simulink model "Clutchless_P2_Parallel_ETE"  (R2017b)
settings: Solver=FixedStepAuto  StartTime=0.0  StopTime=length(Speed)  FixedStep=0.01  MaxStep=0.01  RelTol=1e-3  EnableMultiTasking=on
PostLoadFcn:
  | , if any(exist('dsrtsu_mdlpostloadfcn', 'file') == [2, 3, 6]), try dsrtsu_mdlpostloadfcn('Execute', bdroot); catch fprintf('Error in PostLoadFcn (dsrtsu_mdlpostloadfcn) for model "%s":\n %s\n', bdroot, lasterr); end, end,
undefined symbols (not defined in the file): ABSEnable, Actuators, air, APP1_OOR, APP2_OOR, APP_Mismatch, Brk_Flt, cal, ClutchEngag, Clutchless_HSC_ETE, CS_On_Control, Driver, eng, Engine, EngOverTemp, ENGTRQ_MSMCH_Degraded_CP, ENGTRQ_MSMCH_ErrCritical_CP, ENGTRQ_MSMCH_LimpHome_CP, EngTrqMismatch, env, ess, ESSOverTemp, gb, KeyPos_Flt, KeyPosition, lib_Actuators, lib_Clutchless_HSC_ETE, lib_Driver, lib_EMachine_2017a, lib_Sensors_2017a, LossCAN, Machine, max_vehicle_rad_air_flow, MCUOverTemp, mot, MotDirMismatch, MotOverTemp, MotTrqMismatch, mph2ms, PRNDL_Flt, RegenBrkDisable, RegenFault, Sensors, ShiftLeverPosition, Speed, SW_CS_ON, SW_Engine_ON, t_amb, time, tloop
libraries: simulink x97, Pneumatic_lib x11, nesl_utility x9, EC2_libraries x7, powerlib_meascontrol x2, CalculationGallon x1, lib_Chassis x1, lib_DCDC x1, lib_Differential x1, lib_HVESS x1, fl_lib x1, lib_OBC x1
(part 9 of 9)

== stateflow chart Clutchless_P2_Parallel_ETE/Camaro Plant Model/ICE Simple1/Engine Plant Modified/Core Engine/Crank Process ==
  state Starter_Crank
    du:
    EngActTrq = function(EngSpd_RPM);
  state Eng_Off
    du:
    EngActTrq = 0;
  state Eng_Combustion
    du:
    EngActTrq = 100;
  state CrankTrq = function(EngSpd) [function]
  state Eng_Run
    du:
    EngActTrq = EngBrkTrq;
  (default) -> Eng_Off
  Eng_Off -> Starter_Crank : [EngCrankCmd]
  Starter_Crank -> Eng_Off [order 2] : [!EngCrankCmd]
  Eng_Run -> Eng_Off : [AvlblFuel <= 0.01|| EngShutdown == 1]
  Starter_Crank -> Eng_Combustion [order 1] : [AvlblFuel >= 0.1]
  Eng_Combustion -> Eng_Run : [EngRunAtv]
  data: CrankTrq function_output; EngSpd function_input; EngRunAtv input boolean; AvlblFuel input double; EngActTrq output double; EngCrankCmd input boolean; EngBrkTrq input double; EngSpd_RPM input double; EngShutdown input boolean

== stateflow chart Clutchless_P2_Parallel_ETE/Camaro Plant Model/ICE Simple1/Soft ECM/ECM_RollingAliveCnt/Rolling Alive Counter ==
  state RollingAliveCounter
    state Count1
      en: RollingAliveCnt = 0;
    state Count2
      en: RollingAliveCnt = 1;
    state Count3
      en: RollingAliveCnt = 2;
    state Count4
      en: RollingAliveCnt = 3;
    (default) -> Count1
    Count4 -> Count1 : after(0.01,sec)
    Count1 -> Count2 : after(0.01,sec)
    Count2 -> Count3 : after(0.01,sec)
    Count3 -> Count4 : after(0.01,sec)
  data: RollingAliveCnt output int8 =0

== stateflow chart Clutchless_P2_Parallel_ETE/Camaro Plant Model/ICE Simple1/Soft ECM/Logic ==
  state Eng_Crank
    en:
    EngCrankCmd = 1;
    FuelPumpEnable = 1;
    EngShutdown = 0;
  state Eng_Off
    en:
    EngRunAtv = 0;
    EngCrankCmd = 0;
    ThrottleCmd = 0;
    FuelPumpEnable = 0;
  state Eng_On
    en:
    EngRunAtv = 1;
    EngCrankCmd = 0;
    du:
    ThrottleCmd = APP2TP(drvAPP,EngSpd_RPM);
  state TP = APP2TP(APP,EngSpd) [function]
  (default) -> Eng_Off
  Eng_Off -> Eng_Crank : [SysPwrMd == 3]
  Eng_Crank -> Eng_Off [order 2] : [SysPwrMd < 3]
  Eng_On -> Eng_Off : [SysPwrMd < 2 || EngSpd_RPM < 500]
      | {EngShutdown = 1; }
  Eng_Crank -> Eng_On [order 1] : [EngSpd_RPM >= 580]
  data: TP function_output; APP function_input; EngSpd function_input; drvAPP input; ThrottleCmd output double; EngCrankCmd output boolean; SysPwrMd input int8; ShftLvrPos input int8; EngSpd_RPM input double; VehSpdAvgDrvn input double; EngRunAtv output boolean; FuelPumpEnable output double; EngShutdown output boolean

== stateflow chart Clutchless_P2_Parallel_ETE/Clutchless_HSC_ETE/HSC/Powertrain Manager/HV Manager1/Inverter Manager/MCU_Manager  ==
  state MCU_Initialization
    state MCU_Request_Standby
      en:
      MCU_State = 1;
      RequestedStateINV = 3;
      CAN_Activation = 1;
    state Power_Off_INVCON
      entry:
      MCU_State = 0;
      INVCON_Power =0;
    state Power_On_INVCON
      en:MCU_State = 2;
      INVCON_Power =1;
    state HV_CAN_Actuation_Fault
      en:
      MCU_State = -1;
      CAN_Activation = 0;
    state INVCON_Power_Fault
      en:
      MCU_State = -2;
      INVCON_Power =0;
      CAN_Activation = 0;
    Power_Off_INVCON -> (junction 18) : {Timer=0;}
    (junction 18) -> MCU_Request_Standby [order 1] : [HVCAN_State]
    HV_CAN_Actuation_Fault -> (junction 18) : [HVCAN_State]
    (junction 18) -> HV_CAN_Actuation_Fault [order 2] : after(3,sec)
    (default) -> Power_Off_INVCON
    MCU_Request_Standby -> Power_On_INVCON : [HV_State == 9]
    Power_On_INVCON -> INVCON_Power_Fault : after(3,sec)
        | [INV_State ~= 3]
  state MCU_TorqueMode
    state MCU_Enable
      en:MCU_State = 4;
      RequestedStateINV = 8;
      during: Timer = Timer + 1;
    state MCU_Ready
      en:
      MCU_State = 3;
    state MCU_Running
      en:
      MCU_State =5;
    state TorqueCommand_Reject_Fault
      en:
      MCU_State = -3;
      RequestedStateINV = 3;
    state MCU_Stop
      en:
      MCU_State = 6;
      RequestedStateINV = 3;
    (default) -> MCU_Ready
    MCU_Enable -> (junction 35)
    (junction 35) -> MCU_Running [order 1] : [INV_State == 8]
    MCU_Ready -> MCU_Enable : [EnableInverter]
        | {Timer = 0;}
    (junction 35) -> TorqueCommand_Reject_Fault [order 2] : after(10,sec)
    MCU_Running -> MCU_Stop : [~ReadyToDrive]
  state MCU_Shutdown
    state MCU_Off
      en:
      MCU_State = 11;
      RequestedStateINV = 3;
      INVCON_Power = 0;
    state MCU_Dschrg
      en:
      MCU_State = 10;
      RequestedStateINV = 14;
    state MCU_RdyForShtDwn
      en:
      MCU_State = 9;
    (default) -> MCU_RdyForShtDwn
    MCU_RdyForShtDwn -> MCU_Dschrg : [~EnableInverter]
        | {Timer = 0;}
    MCU_Dschrg -> MCU_Off : [INV_State == 14 && LinkVoltage<60]
  (default) -> MCU_Initialization
  MCU_Shutdown -> MCU_Initialization : [KeyPos>= 1]
  MCU_Initialization -> MCU_Shutdown [order 2] : [ReadyToCharge]
  MCU_TorqueMode -> MCU_Initialization [order 1] : [INV_State == 14]
  MCU_Initialization -> MCU_TorqueMode [order 1] : [INV_State == 3 && INVCON_Power_Feedback && ReadyToDrive]
  MCU_TorqueMode -> MCU_Shutdown [order 2] : [INV_State == 3 && ~ReadyToDrive]
  data: ReadyToDrive input boolean; ReadyToCharge input; HV_State input; HVCAN_State input boolean; INVCON_Power_Feedback input; KeyPos input; LinkVoltage input; INV_State input; INV_CurrentHV input; Timer local double; MCU_State output; EnableInverter input boolean; ShutdownCurrent input; INVCON_Power output double; RequestedStateINV output; CAN_Activation output

== matlab function Clutchless_P2_Parallel_ETE/Camaro Plant Model/E-Machine/Soft MCU/diff_INV_state1 ==
  data: u input; y output
function y = fcn(u)
if(u == 0) %when inverter is in standby state
    y = 0;
elseif(u == 1) %when inverter is in torque control state
    y = 1;
elseif(u==2) %when invertor is in error state
    y = 0;
else
    y = 0;
end

== stateflow chart Clutchless_P2_Parallel_ETE/Clutchless_HSC_ETE/HSC/Camaro Fault Detection/Signal Diagnostic/ESS Signal Diagnostic/ESS SOC Validity Check/essSOC_0_1Range ==
  state aboveMax
    en: essSOCRange=3;
  state NormalRange
    en: essSOCRange=2;
  state LowRange
    en:essSOCRange=1;
  state BelowNormal
    en: essSOCRange=0;
  aboveMax -> NormalRange : [signalValue<0.95]
  NormalRange -> aboveMax [order 1] : [signalValue>=0.95]
  NormalRange -> NormalRange [order 3] : [clearFaults==1]
      | {essSOCRange=2;}
  (default) -> NormalRange
  LowRange -> NormalRange [order 1] : [signalValue>0.3]
  NormalRange -> LowRange [order 2] : [signalValue<=0.3&&signalValue>0.15]
  LowRange -> BelowNormal [order 2] : [signalValue<=0.15]
  BelowNormal -> LowRange : [signalValue>0.15]
  data: clearFaults input; signalValue input; data local; essSOCRange output

== stateflow chart Clutchless_P2_Parallel_ETE/Clutchless_HSC_ETE/HSC/Camaro Fault Detection/Signal Diagnostic/ESS Signal Diagnostic/ESS Temp Validity Check/essTsignalRange ==
  state AboveMax
    en: essTempRange=4;
  state HighRange
    en: essTempRange=3;
  state NormalRange
    en: essTempRange=2;
  state LowRange
    en:essTempRange=1;
  state BelowNormal
    en: essTempRange=0;
  HighRange -> AboveMax [order 2] : [signalValue>55]
  AboveMax -> HighRange : [signalValue<55]
  HighRange -> NormalRange [order 1] : [signalValue<=30]
  NormalRange -> HighRange [order 1] : [signalValue>32]
  NormalRange -> NormalRange [order 3] : [clearFaults==1]
      | {essTempRange=2;}
  (default) -> NormalRange
  LowRange -> NormalRange [order 1] : [signalValue>=30]
  NormalRange -> LowRange [order 2] : [signalValue<0 ]
  LowRange -> BelowNormal [order 2] : [signalValue<-28]
  BelowNormal -> LowRange : [signalValue>28]
  data: clearFaults input; signalValue input; essTempRange output; data local

== stateflow chart Clutchless_P2_Parallel_ETE/Clutchless_HSC_ETE/HSC/Camaro Fault Detection/Signal Diagnostic/ESS Signal Diagnostic/Rolling Alive Counter Detection/Chart ==
  state Off
    en:flag=0;
  state Alive
    en:flag=1;
  state Dead
    en:flag=0;
  Alive -> Alive [order 1] : after(CycleTime-tloop,sec)
      | [PulseDetect==1]
  (default) -> Off
  Off -> Alive : [PulseDetect==1]
  Alive -> Dead [order 2] : after(CycleTime,sec)
  data: PulseDetect input; CycleTime input; flag output; tloop input

== stateflow chart Clutchless_P2_Parallel_ETE/Clutchless_HSC_ETE/HSC/Camaro Fault Detection/Signal Diagnostic/Engine Signal Diagnostic/Rolling Alive Counter Detection1/Chart ==
  state Off
    en:flag=0;
  state Alive
    en:flag=1;
  state Dead
    en:flag=0;
  Alive -> Alive [order 1] : after(CycleTime-tloop,sec)
      | [PulseDetect==1]
  (default) -> Off
  Off -> Alive : [PulseDetect==1]
  Alive -> Dead [order 2] : after(CycleTime,sec)
  data: PulseDetect input; CycleTime input; flag output; tloop parameter

== stateflow chart Clutchless_P2_Parallel_ETE/Clutchless_HSC_ETE/HSC/Camaro Fault Detection/Signal Diagnostic/Transmission Signal Diagnostic/Rolling Alive Counter Detection/Chart ==
  state Off
    en:flag=0;
  state Alive
    en:flag=1;
  state Dead
    en:flag=0;
  Alive -> Alive [order 1] : after(CycleTime-tloop,sec)
      | [PulseDetect==1]
  (default) -> Off
  Off -> Alive : [PulseDetect==1]
  Alive -> Dead [order 2] : after(CycleTime,sec)
  data: PulseDetect input; CycleTime input; flag output; tloop parameter

== stateflow chart Clutchless_P2_Parallel_ETE/Clutchless_HSC_ETE/HSC/Powertrain Manager/Torque Distribution/Sport Mode Enable/Sports Mode Logic ==
  state Sport_Mode
    entry:
    Driver_Mode=2;
  state Hybrid_Mode
    entry:
    Driver_Mode=1;
  Hybrid_Mode -> Sport_Mode : [Voltage_Input>3.5&&Voltage_Input<3.9]
  (default) -> Hybrid_Mode
  Sport_Mode -> Hybrid_Mode : [Voltage_Input>1.8&&Voltage_Input<2.2]
  data: Voltage_Input input; Driver_Mode output

== stateflow chart Clutchless_P2_Parallel_ETE/Clutchless_HSC_ETE/HSC/Powertrain Manager/Torque Distribution/Supervisory  Control  Logic ==
  note: 
  note: Tranmission Shift Level Position (ShftLvrPos):
  state VehOn
    en:
    mode = 6;
    HV_Req=1;
  state VehOffOrAcc
    en:
    mode=0;
    EnablePrplsn = 0;
    HV_Req=0;
    closeMaincReq=0;
  state Close_Contactors
    en:
    closeMaincReq=1;
  state ChgTrans
    en:
    mode=10;
  state Wait
  state VehShutdown
    en:
    powerMode = 1;
    EnablePrplsn = 0;
    EngOnReq = 0;
    EngAppReq = 0;
    EnableInverter=0;
    mode=8;
  note: System Power Mode (KeyPos):
  state Charging
    en:
    mode = 9;
    HV_Req=1;
    closeMaincReq = 1;
    EnablePrplsn = 0;
    EnableInverter = 0;
  state EnablePropulsion
    en:
    mode=7;
    EnablePrplsn = 1;
    EngOnReq=1;
  state HV_Shutdown
    en:
    HV_Req=0;
    closeMaincReq=0;
  state IMG_Shutdown
    en:
    MotTrqReq = 0;
  state VehReady
    en:
    powerMode = 2;
    state CD_Mode1
      en:
      mode=1;
      EngOnReq=1;
      state Drive_mode
        en:
        Brkmode=0;
        du:
        MotTrqReq = MotTrqCalc2(drvAPP,ShftLvrPos,DrvIntdAxleTrq,TransRatio,EngTrq);
        EngTrq=EngTrqCalc(EngSpd,drvAPP,VehicleSpeed,ShftLvrPos,DrvIntdAxleTrq,TransRatio);
        EngAppReq=EngTrq2EngApp(EngTrq,TransRatio);
        state MotTrq = MotTrqCalc2(APP,ShftLvrPos,DrvIntdAxleTrq,TransRatio,Trq) [function]
        state Trq = EngTrqCalc(EngSpeed,APP,VehSpd,ShftLvrPos,DrvIntdAxleTrq,TransRatio) [function]
        state APP = EngTrq2EngApp(Trq,TransRatio) [function]
      state Brake_mode
        en:
        EngAppReq=0;
        state Regen_mode
          en:
          Brkmode=1;
          du:
          MotTrqReq=MotTrqCalc1(BrkPdlPos,VehicleSpeed,...
          ShftLvrPos,MotSpd,TransRatio,IntdAxleTrq);
        state No_regen
          en:
          Brkmode=2;
          du:
          MotTrqReq=MotTrqCalc2(ShftLvrPos,TransRatio);
        state Temp_delay
        state Temp_delay1
        state T = MotTrqCalc1(BPP,VehSpd,ShftLvrPos,MotSpeed,TransRatio,IntdAxleTrq) [function]
        state T = MotTrqCalc2(ShftLvrPos,TransRatio) [function]
        (default) -> VehReady.CD_Mode1.Brake_mode.No_regen
        VehReady.CD_Mode1.Brake_mode.Regen_mode -> VehReady.CD_Mode1.Brake_mode.Temp_delay : [RegenBrkDisable||SoC>=80||ABSAtv||Regen_fault]
        VehReady.CD_Mode1.Brake_mode.Temp_delay -> VehReady.CD_Mode1.Brake_mode.No_regen : after(0.25,sec)
        VehReady.CD_Mode1.Brake_mode.Temp_delay1 -> VehReady.CD_Mode1.Brake_mode.Regen_mode : after(0.25,sec)
        VehReady.CD_Mode1.Brake_mode.No_regen -> VehReady.CD_Mode1.Brake_mode.Temp_delay1 : [RegenBrkDisable == 0&&SoC<80&&ABSAtv==0&&Regen_fault==0]
      state Time_delay
      state Time_delay1
      (default) -> Drive_mode
      Drive_mode -> Time_delay : [BrkPdlPos>0&&IntdAxleTrq<0]
      Time_delay -> Brake_mode : after(0.25,sec)
      Time_delay1 -> Drive_mode : after(0.25,sec)
      Brake_mode -> Time_delay1 : [drvAPP>0&&IntdAxleTrq>=0]
    state EnableINV2
      en:
      EnableInverter=1
    state EnableINV
      en:
      EnableInverter=1
    state Eng_Charging_Stat
      en:
      EngOnReq = 1;
      mode=5;
      du:
      MotTrqReq = MotTrqCalc(ShftLvrPos,DrvIntdAxleTrq,EngTrq);
      EngTrq = EngTrqCalc(EngSpd,ShftLvrPos,DrvIntdAxleTrq,TransRatio);
      EngAppReq=drvAPP;
      state Trq = EngTrqCalc(EngSpeed,ShftLvrPos,DrvIntdAxleTrq,TransRatio) [function]
      state MotTrq = MotTrqCalc(ShftLvrPos,DrvIntdAxleTrq,Trq) [function]
      state APP = EngTrq2EngApp(Trq,TransRatio) [function]
    state EnableINV1
      en:
      EnableInverter=1
    state CS_Mode
      state Engine_Charge
        en:
        mode=2;
        EngOnReq=1;
        state Eng_Charge_CS
          du:
          MotTrqReq = MotTrqCalc(ShftLvrPos,DrvIntdAxleTrq,EngTrq,SoC,Voltage);
          EngTrq = EngTrqCalc(drvAPP,EngSpd,ShftLvrPos,DrvIntdAxleTrq,TransRatio);
          EngAppReq=EngTrq2EngApp(EngTrq,TransRatio);
          state Trq = EngTrqCalc(APP,EngSpeed,ShftLvrPos,DrvIntdAxleTrq,TransRatio) [function]
          state MotTrq = MotTrqCalc(ShftLvrPos,DrvIntdAxleTrq,Trq,SoC,Volt) [function]
          state APP = EngTrq2EngApp(Trq,TransRatio) [function]
        state Brake_mode1
          en:
          EngAppReq=0.51;
          state No_regen
            en:
            Brkmode=2;
            du:
            MotTrqReq=MotTrqCalc2(ShftLvrPos,TransRatio);
          state Regen_mode
            en:
            Brkmode=1;
            du:
            MotTrqReq=MotTrqCalc1(BrkPdlPos,VehicleSpeed,...
            ShftLvrPos,MotSpd,TransRatio,IntdAxleTrq);
          state Temp_delay
          state Temp_delay1
          state T = MotTrqCalc1(BPP,VehSpd,ShftLvrPos,MotSpeed,TransRatio,IntdAxleTrq) [function]
          state T = MotTrqCalc2(ShftLvrPos,TransRatio) [function]
          (default) -> VehReady.CS_Mode.Engine_Charge.Brake_mode1.No_regen
          VehReady.CS_Mode.Engine_Charge.Brake_mode1.Regen_mode -> VehReady.CS_Mode.Engine_Charge.Brake_mode1.Temp_delay : [RegenBrkDisable||SoC>=80||ABSAtv||Regen_fault]
          VehReady.CS_Mode.Engine_Charge.Brake_mode1.Temp_delay -> VehReady.CS_Mode.Engine_Charge.Brake_mode1.No_regen : after(0.25,sec)
          VehReady.CS_Mode.Engine_Charge.Brake_mode1.Temp_delay1 -> VehReady.CS_Mode.Engine_Charge.Brake_mode1.Regen_mode : after(0.25,sec)
          VehReady.CS_Mode.Engine_Charge.Brake_mode1.No_regen -> VehReady.CS_Mode.Engine_Charge.Brake_mode1.Temp_delay1 : [RegenBrkDisable == 0&&EngSpd>1000&&SoC<80&&ABSAtv==0&&Regen_fault==0]
        state Time_delay3
        state Time_delay2
        (default) -> Eng_Charge_CS
        Eng_Charge_CS -> Time_delay3 : [BrkPdlPos>0 && IntdAxleTrq<0]
        Time_delay3 -> Brake_mode1 : after(0.25,sec)
        Brake_mode1 -> Time_delay2 : [drvAPP>0&&IntdAxleTrq>=0]
        Time_delay2 -> Eng_Charge_CS : after(0.25,sec)
      (default) -> Engine_Charge
    (default) -> (junction 1935)
    (junction 1935) -> EnableINV2 [order 2] : [!SW_CS_ON&&...
        | CDmode==0&&SW_Engine_ON...
        | &&ShftLvrPos==1&&HoodStatus==0]
    (junction 1935) -> EnableINV [order 1] : [CDmode==1&&!SW_Engine_ON...
        | &&!SW_CS_ON]
    EnableINV -> CD_Mode1 : [INV_State==8]
    EnableINV2 -> Eng_Charging_Stat : [INV_State==8]
    (junction 1935) -> EnableINV1 [order 3] : [SW_CS_ON&&...
        | CDmode==0&&!SW_Engine_ON]
    CD_Mode1 -> CS_Mode : [(SW_CS_ON&&...
        | CDmode==0&&!SW_Engine_ON)||SoC<CS_SOC_MIN]
    EnableINV1 -> CS_Mode : [INV_State==8]
  VehOffOrAcc -> EnablePropulsion [order 2] : [KeyPos==3&&BrkPdlPos>10&&ShftLvrPos==1&&(~eSystemStatus&&iceSystemStatus)]
  VehOffOrAcc -> VehOn [order 1] : [KeyPos>= 1&&(eSystemStatus||iceSystemStatus)]
  VehOn -> VehOffOrAcc [order 2] : [KeyPos<1]
  VehOn -> Close_Contactors [order 1] : [InverterEnabled==3]
  (default) -> VehOffOrAcc
  Close_Contactors -> VehOffOrAcc [order 3] : [KeyPos<1]
  ChgTrans -> VehOffOrAcc [order 2] : [plugged==0]
  VehOffOrAcc -> ChgTrans [order 3] : [plugged]
      | {HV_Req=1;}
  Close_Contactors -> Charging [order 2] : [plugged]
  VehShutdown -> VehOffOrAcc [order 2] : after(1,sec)...
      | [plugged==0]
  Wait -> VehOffOrAcc [order 1] : after(3,sec)...
      | [plugged==0]
  ChgTrans -> Charging [order 1] : after(4,sec)...
      | [INV_State==3]
  Close_Contactors -> EnablePropulsion [order 1] : [KeyPos==3&&BrkPdlPos>10&&...
      | ShftLvrPos==1]
  Charging -> Wait : [plugged==0]
  Wait -> Charging [order 2] : after(3,sec)...
      | [plugged==1]
  VehShutdown -> Charging [order 1] : [plugged]
  HV_Shutdown -> VehShutdown : [InverterEnabled==3]
  EnablePropulsion -> Charging [order 2] : [plugged]
  EnablePropulsion -> VehReady [order 1] : after(0.5,sec)
  VehReady -> Charging [order 1] : [plugged]
  IMG_Shutdown -> HV_Shutdown : [MotSpd<10&&ShftLvrPos==1]
  VehReady -> IMG_Shutdown [order 2] : [KeyPos < 2 ...
      | ||(eSystemStatus==0&&...
      | iceSystemStatus==0)]
  data: APP function_input; MotTrq function_output; ShftLvrPos function_input; DrvIntdAxleTrq function_input; TransRatio function_input; Trq function_input; Trq function_output; EngSpeed function_input; APP function_input; VehSpd function_input; ShftLvrPos function_input; DrvIntdAxleTrq function_input; TransRatio function_input; Trq function_input; APP function_output; TransRatio function_input; T function_output; BPP function_input; VehSpd function_input; ShftLvrPos function_input; MotSpeed function_input; TransRatio function_input; IntdAxleTrq function_input; T function_output; ShftLvrPos function_input; TransRatio function_input; Trq function_output; EngSpeed function_input; ShftLvrPos function_input; DrvIntdAxleTrq function_input; TransRatio function_input; MotTrq function_output; ShftLvrPos function_input; DrvIntdAxleTrq function_input; Trq function_input; Trq function_input; APP function_output; TransRatio function_input; APP function_input; Trq function_output; EngSpeed function_input; ShftLvrPos function_input; DrvIntdAxleTrq function_input; TransRatio function_input; MotTrq function_output; ShftLvrPos function_input; DrvIntdAxleTrq function_input; Trq function_input; SoC function_input; Volt function_input; Trq function_input; APP function_output; TransRatio function_input; T function_output; BPP function_input; VehSpd function_input; ShftLvrPos function_input; MotSpeed function_input; TransRatio function_input; IntdAxleTrq function_input; T function_output; ShftLvrPos function_input; TransRatio function_input; data local double; SportModeEnabled input boolean; TransEstGear input int8; mode output int8; powerMode output int8; closeMaincReq output double; EnablePrplsn output boolean; KeyPos input int8; BrkPdlPos input double; drvAPP input double; VehicleSpeed input double; EngSpd input double; MotSpd input double; ShftLvrPos input int8; EngAppReq output double; EngOnReq output boolean; MotTrqReq output double; EnableInverter output boolean; InverterEnabled input double; plugged input double; CD_SOC_MIN input double; CS_SOC_MIN input double; CS_SOC_MAX input double; EngRunAtv input boolean; SoC input double; EngTrq output double; DrvIntdAxleTrq input double; IntdAxleTrq input double; Faked_SoC input double; TransRatio input double; HV_Req output double; SW_CS_ON input boolean; SW_Engine_ON input boolean; RegenBrkDisable input boolean; Chg output double; Brkmode output double; Drvmode output double; eSystemStatus input; iceSystemStatus input; Drv_Mode local double; ABSAtv input boolean; Regen_fault input boolean; EngFdbkTrq input double; EngCtlTmp input; ClutchEngage output double; INV_State input; HoodStatus input; CDmode input; Voltage input

== stateflow chart Clutchless_P2_Parallel_ETE/Clutchless_HSC_ETE/HSC/Camaro Fault Detection/Component Diagnostic/Transmission Component Diagnostic/TCM_CompDia ==
  state TCM_Offline
    en: TCM_Status=0;
  state TCM_Limited [commented out]
    en: TCM_Status=1;
  state TCM_Online
    en: TCM_Status=2;
  (default) -> TCM_Offline
  TCM_Online -> TCM_Offline : [~TCMRollingAliveActive_SigValid||...
      | ~LvrPosTrnsShft_SigValid||...
      | ~TransEstGear_SigValid||...
      | ~LockupCmd_SigValid||VehDirFault]
  TCM_Offline -> TCM_Online : [TCMRollingAliveActive_SigValid&&...
      | LvrPosTrnsShft_SigValid&&TransEstGear_SigValid&&...
      | LockupCmd_SigValid&&VehDirFault==0]
  TCM_Online -> TCM_Limited [commented out]
  TCM_Limited -> TCM_Online [commented out]
  data: TCM_Status output; TCMRollingAliveActive_SigValid input; LvrPosTrnsShft_SigValid input; TransEstGear_SigValid input; LockupCmd_SigValid input; VehDirFault input

== stateflow chart Clutchless_P2_Parallel_ETE/Clutchless_HSC_ETE/HSC/Camaro Fault Detection/Input Conversions/TCM_Conversions/TCM_RollinAliveCounter/Rolling Alive Counter1 ==
  state RollingAliveCounter
    state Count1
      en: RollingAliveCnt=0;
    state Count2
      en: RollingAliveCnt=1;
    state Count3
      en: RollingAliveCnt=2;
    state Count4
      en: RollingAliveCnt=3;
    (default) -> Count1
    Count4 -> Count1 : after(0.01,sec)
    Count1 -> Count2 : after(0.01,sec)
    Count2 -> Count3 : after(0.01,sec)
    Count3 -> Count4 : after(0.01,sec)
  data: RollingAliveCnt output double

== stateflow chart Clutchless_P2_Parallel_ETE/Clutchless_HSC_ETE/HSC/Camaro Fault Detection/Signal Diagnostic/Engine Signal Diagnostic/Engine_Temp[DegC] ==
  state AboveMax
    en: EngTempRange=3;
  state HighRange
    en: EngTempRange=2;
  state NormalRange
    en: EngTempRange=1;
  HighRange -> AboveMax [order 2] : [Engine_Temp_DegC>120]
  AboveMax -> HighRange : [Engine_Temp_DegC<120]
  NormalRange -> HighRange [order 1] : [Engine_Temp_DegC>100&&Engine_Temp_DegC<120]
  HighRange -> NormalRange [order 1] : [Engine_Temp_DegC<=100]
  NormalRange -> NormalRange [order 2] : [clearFaults==1]
      | {EngTempRange=1;}
  (default) -> NormalRange
  data: clearFaults input; Engine_Temp_DegC input; EngTempRange output; data local

== stateflow chart Clutchless_P2_Parallel_ETE/Clutchless_HSC_ETE/HSC/Powertrain Manager/Thermal Manager/ESS Pump Manger/Chart1 ==
  state ESS_Pump [parallel]
    settings: executionOrder=1
    state pump_state_0
      entry: ESS_pump_control=0;
    state pump_low_State_1
      entry: ESS_pump_control=30;
    state pump_transition_3_to_0
    state pump_transition_2_to_0
    state pump_high_State_3
      entry: ESS_pump_control=90;
    state pump_medi_State_2
      entry: ESS_pump_control=60;
    pump_state_0 -> pump_low_State_1 : [(ESS_temp>=ESS_Temp_State_1_Thrs)&&SysPowMod>0]
    (default) -> pump_state_0
    pump_low_State_1 -> pump_state_0 [order 1] : [(ESS_temp<ESS_Temp_State_1_Thrs&&after(10,sec))||SysPowMod==0 ]
    pump_transition_2_to_0 -> pump_state_0 : after(15,sec)
    pump_transition_3_to_0 -> pump_state_0 : after(30,sec)
    pump_low_State_1 -> pump_medi_State_2 [order 2] : [ESS_temp>=ESS_Temp_State_2_Thrs]
    pump_medi_State_2 -> pump_low_State_1 [order 1] : [ESS_temp<ESS_Temp_State_2_Thrs&&after(10,sec)]
    pump_high_State_3 -> pump_transition_3_to_0 [order 2] : [SysPowMod==0]
    pump_medi_State_2 -> pump_transition_2_to_0 [order 3] : [SysPowMod==0]
    pump_medi_State_2 -> pump_high_State_3 [order 2] : [ESS_temp>=ESS_Temp_State_3_Thrs]
    pump_high_State_3 -> pump_medi_State_2 [order 1] : [ESS_temp<ESS_Temp_State_3_Thrs&&after(10,sec)]
  state ESS_comp [parallel]
    settings: executionOrder=2
    state Comp_off
      entry:
      ESS_comp=0;
      ESS_val=0;
      ESS_comp_Enable = 1;
    state Comp_on
      entry:
      ESS_comp=10;
      ESS_val=1;
      ESS_comp_Enable = 0;
    (default) -> Comp_off
    Comp_off -> Comp_on : [(ESS_CltTemp>=ESS_Comp_TempThrs)&&SysPowMod>0]
    Comp_on -> Comp_off : [(ESS_CltTemp<ESS_Comp_TempThrs&&after(25,sec))&&SysPowMod==0]
  data: ESS_temp input; ESS_comp output; ESS_pump_control output; ESS_val output; ESS_Temp_State_1_Thrs input double =15; ESS_Temp_State_2_Thrs input double; ESS_Temp_State_3_Thrs input double; ESS_Comp_TempThrs input double; ESS_CltTemp input; ESS_comp_Enable output; SysPowMod input

== stateflow chart Clutchless_P2_Parallel_ETE/Clutchless_HSC_ETE/HSC/Powertrain Manager/Thermal Manager/MotInv Pump Manger/MCUPump_Manager ==
  state Pump_Off
    entry: MotInvpump_control=0;
  state Pump_transition_2_to_off
  state Pump_High_State_2
    entry: MotInvpump_control=90;
  state Pump_Low_State_1
    entry: MotInvpump_control=60;
  (default) -> Pump_Off
  Pump_transition_2_to_off -> Pump_Off : after(30,sec)
  Pump_Off -> Pump_Low_State_1 : [(Motor_temp>=Mot_Temp_State_1_Thrs||MCU_temp>=MCU_Temp_State_1_Thrs)&&after(10,sec)&&SysPowMod>0]
  Pump_Low_State_1 -> Pump_Off [order 2] : [((Motor_temp<Mot_Temp_State_1_Thrs)&&(MCU_temp<MCU_Temp_State_1_Thrs)&&after(10,sec))||SysPowMod==0]
  Pump_High_State_2 -> Pump_transition_2_to_off [order 2] : [SysPowMod==0]
  Pump_Low_State_1 -> Pump_High_State_2 [order 1] : [(Motor_temp>=Mot_Temp_State_2_Thrs||MCU_temp>=MCU_Temp_State_2_Thrs)&&after(10,sec)]
  Pump_High_State_2 -> Pump_Low_State_1 [order 1] : [(Motor_temp<Mot_Temp_State_2_Thrs&&MCU_temp<MCU_Temp_State_2_Thrs)&&(after(10,sec))]
  data: MotInvpump_control output; Motor_temp input; MCU_temp input; MCU_Temp_State_1_Thrs input double; Mot_Temp_State_1_Thrs input double; MCU_Temp_State_2_Thrs input double; Mot_Temp_State_2_Thrs input double; SysPowMod input
